simulink model "TST_InjCtl_qCo"  (R2016b)
settings: Solver=FixedStepDiscrete  StartTime=0.0  StopTime=simTime  FixedStep=sampleTime  RelTol=1e-3
values from neighbouring files (symbols this model uses):
  testCase = 1    [initTST_InjCtl_qCo_001.m]    (also in initTST_InjCtl_qCo_002.m = 2; initTST_InjCtl_qCo_003.m = 3; initTST_InjCtl_qCo_004.m = 4)
libraries: simulink x9, UnitTest_Lib x6
settings Model: Creator=zhengjinyan  LastModifiedBy=zhengjinyan
settings DebuggingCC: SignalRangeChecking=error

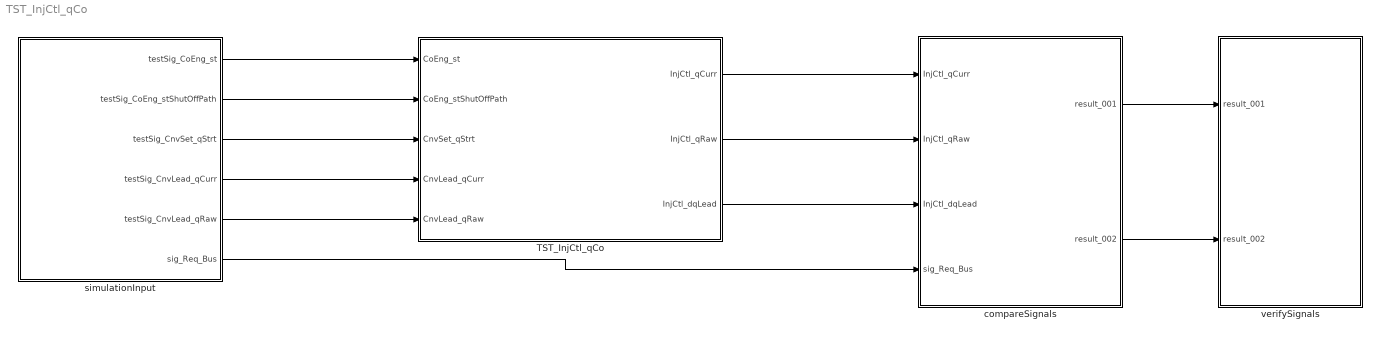
== system TST_InjCtl_qCo ==
  TST_InjCtl_qCo : Subsystem
  compareSignals : Subsystem
  simulationInput : Subsystem
  verifySignals : Subsystem
  wires:
  simulationInput/1(testSig_CoEng_st) -> TST_InjCtl_qCo/1(CoEng_st)
  simulationInput/2(testSig_CoEng_stShutOffPath) -> TST_InjCtl_qCo/2(CoEng_stShutOffPath)
  simulationInput/3(testSig_CnvSet_qStrt) -> TST_InjCtl_qCo/3(CnvSet_qStrt)
  simulationInput/4(testSig_CnvLead_qCurr) -> TST_InjCtl_qCo/4(CnvLead_qCurr)
  simulationInput/5(testSig_CnvLead_qRaw) -> TST_InjCtl_qCo/5(CnvLead_qRaw)
  TST_InjCtl_qCo/1(InjCtl_qCurr) -> compareSignals/1(InjCtl_qCurr)
  TST_InjCtl_qCo/2(InjCtl_qRaw) -> compareSignals/2(InjCtl_qRaw)
  TST_InjCtl_qCo/3(InjCtl_dqLead) -> compareSignals/3(InjCtl_dqLead)
  simulationInput/6(sig_Req_Bus) -> compareSignals/4(sig_Req_Bus)
  compareSignals/1(result_001) -> verifySignals/1(result_001)
  compareSignals/2(result_002) -> verifySignals/2(result_002)

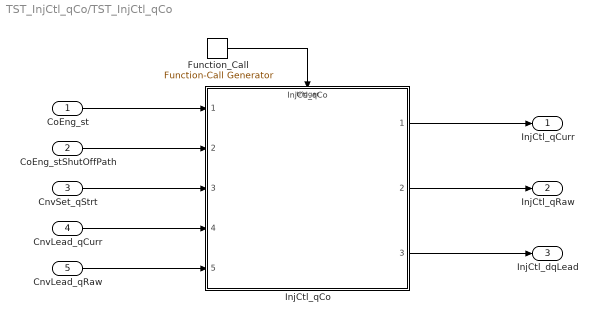
== system TST_InjCtl_qCo/TST_InjCtl_qCo ==
  CoEng_st : Inport
  CoEng_stShutOffPath : Inport  Port=2
  CnvSet_qStrt : Inport  Port=3
  CnvLead_qCurr : Inport  Port=4
  CnvLead_qRaw : Inport  Port=5
  Function_Call : simulink/Ports & Subsystems/Function-Call Generator  sample_time=sampleTime  numberOfIterations=1
  InjCtl_qCo : ModelReference  ModelNameDialog=InjCtl_qCo  SimulationMode=Normal  ModelReferenceVersion=1.10  TriggerPortName=function  TriggerPortTriggerType=function-call  TriggerPortStatesWhenEnabling=held
  InjCtl_qCurr : Outport
  InjCtl_qRaw : Outport  Port=2
  InjCtl_dqLead : Outport  Port=3
  wires:
  Function_Call/1 -> InjCtl_qCo/Trigger
  CoEng_st/1 -> InjCtl_qCo/1
  CoEng_stShutOffPath/1 -> InjCtl_qCo/2
  CnvSet_qStrt/1 -> InjCtl_qCo/3
  CnvLead_qCurr/1 -> InjCtl_qCo/4
  CnvLead_qRaw/1 -> InjCtl_qCo/5
  InjCtl_qCo/1 -> InjCtl_qCurr/1
  InjCtl_qCo/2 -> InjCtl_qRaw/1
  InjCtl_qCo/3 -> InjCtl_dqLead/1

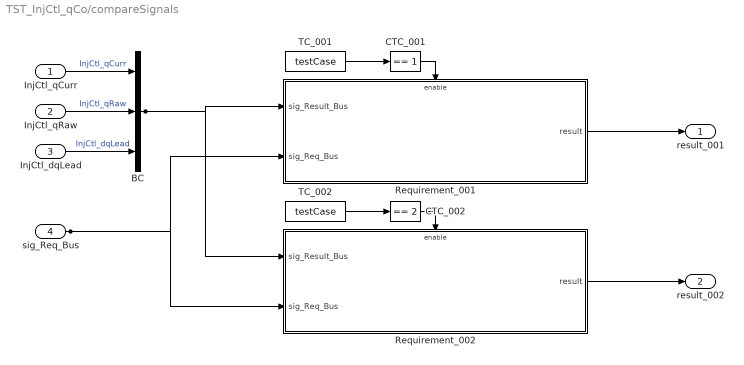
== system TST_InjCtl_qCo/compareSignals ==
  InjCtl_qCurr : Inport
  InjCtl_qRaw : Inport  Port=2
  InjCtl_dqLead : Inport  Port=3
  sig_Req_Bus : Inport  Port=4
  BC : BusCreator  Inputs=3
  CTC_001 : simulink/Logic and Bit Operations/Compare To Constant  relop===  const=1  OutDataTypeStr=boolean
  CTC_002 : simulink/Logic and Bit Operations/Compare To Constant  relop===  const=2  OutDataTypeStr=boolean
  Requirement_001 : Subsystem
  Requirement_002 : Subsystem
  TC_001 : Constant  Value=testCase
  TC_002 : Constant  Value=testCase
  result_001 : Outport
  result_002 : Outport  Port=2
  wires:
  InjCtl_qCurr/1 -> BC/1  "InjCtl_qCurr"
  InjCtl_qRaw/1 -> BC/2  "InjCtl_qRaw"
  InjCtl_dqLead/1 -> BC/3  "InjCtl_dqLead"
  TC_001/1 -> CTC_001/1
  CTC_001/1 -> Requirement_001/Enable
  sig_Req_Bus/1 -> Requirement_001/2(sig_Req_Bus), Requirement_002/2(sig_Req_Bus)
  BC/1 -> Requirement_001/1(sig_Result_Bus), Requirement_002/1(sig_Result_Bus)
  Requirement_001/1(result) -> result_001/1
  TC_002/1 -> CTC_002/1
  CTC_002/1 -> Requirement_002/Enable
  Requirement_002/1(result) -> result_002/1

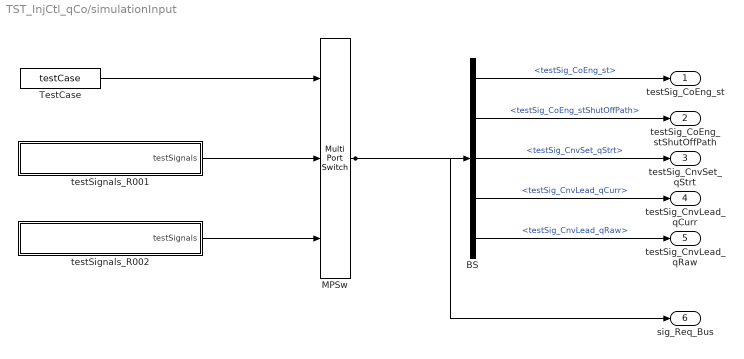
== system TST_InjCtl_qCo/simulationInput ==
  BS : BusSelector  OutputSignals=testSig_CoEng_st,testSig_CoEng_stShutOffPath,testSig_CnvSet_qStrt,testSig_CnvLead_qCurr,testSig_CnvLead_qRaw
  MPSw : MultiPortSwitch  Inputs=2  SaturateOnIntegerOverflow=on  InputSameDT=on
  TestCase : Constant  Value=testCase
  testSignals_R001 : Subsystem
  testSignals_R002 : Subsystem
  testSig_CoEng_st : Outport
  testSig_CoEng_stShutOffPath : Outport  Port=2
  testSig_CnvSet_qStrt : Outport  Port=3
  testSig_CnvLead_qCurr : Outport  Port=4
  testSig_CnvLead_qRaw : Outport  Port=5
  sig_Req_Bus : Outport  Port=6
  wires:
  BS/1 -> testSig_CoEng_st/1  "<testSig_CoEng_st>"
  BS/2 -> testSig_CoEng_stShutOffPath/1  "<testSig_CoEng_stShutOffPath>"
  BS/3 -> testSig_CnvSet_qStrt/1  "<testSig_CnvSet_qStrt>"
  BS/4 -> testSig_CnvLead_qCurr/1  "<testSig_CnvLead_qCurr>"
  BS/5 -> testSig_CnvLead_qRaw/1  "<testSig_CnvLead_qRaw>"
  MPSw/1 -> BS/1, sig_Req_Bus/1
  TestCase/1 -> MPSw/1
  testSignals_R001/1(testSignals) -> MPSw/2
  testSignals_R002/1(testSignals) -> MPSw/3

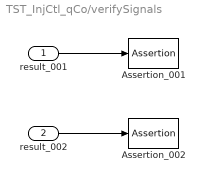
== system TST_InjCtl_qCo/verifySignals ==
  result_001 : Inport
  result_002 : Inport  Port=2
  Assertion_001 : Assertion  Enabled=off
  Assertion_002 : Assertion  Enabled=off
  wires:
  result_001/1 -> Assertion_001/1
  result_002/1 -> Assertion_002/1

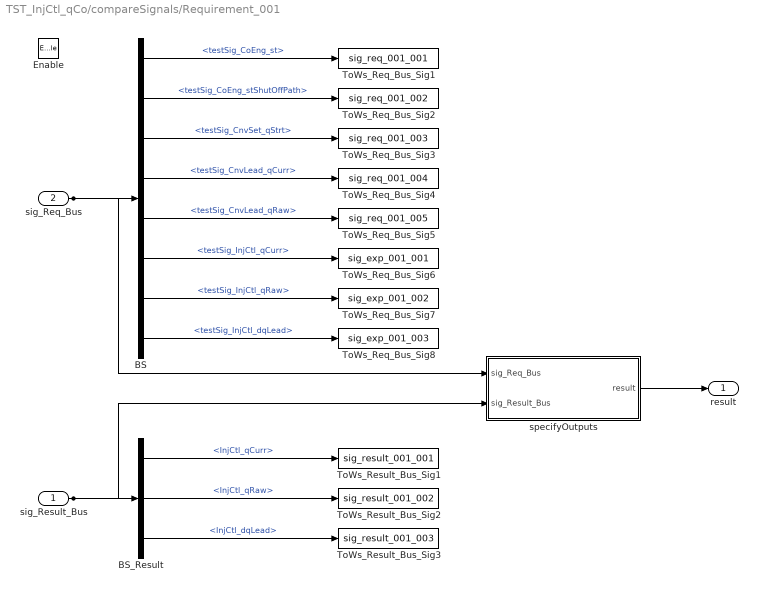
== system TST_InjCtl_qCo/compareSignals/Requirement_001 ==
  sig_Result_Bus : Inport
  sig_Req_Bus : Inport  Port=2
  Enable : EnablePort
  BS : BusSelector  OutputSignals=testSig_CoEng_st,testSig_CoEng_stShutOffPath,testSig_CnvSet_qStrt,testSig_CnvLead_qCurr,testSig_CnvLead_qRaw,testSig_InjCtl_qCurr,testSig_InjCtl_qRaw,testSig_InjCtl_dqLead
  BS_Result : BusSelector  OutputSignals=InjCtl_qCurr,InjCtl_qRaw,InjCtl_dqLead
  ToWs_Req_Bus_Sig1 : ToWorkspace  VariableName=sig_req_001_001  SaveFormat=Structure With Time
  ToWs_Req_Bus_Sig2 : ToWorkspace  VariableName=sig_req_001_002  SaveFormat=Structure With Time
  ToWs_Req_Bus_Sig3 : ToWorkspace  VariableName=sig_req_001_003  SaveFormat=Structure With Time
  ToWs_Req_Bus_Sig4 : ToWorkspace  VariableName=sig_req_001_004  SaveFormat=Structure With Time
  ToWs_Req_Bus_Sig5 : ToWorkspace  VariableName=sig_req_001_005  SaveFormat=Structure With Time
  ToWs_Req_Bus_Sig6 : ToWorkspace  VariableName=sig_exp_001_001  SaveFormat=Structure With Time
  ToWs_Req_Bus_Sig7 : ToWorkspace  VariableName=sig_exp_001_002  SaveFormat=Structure With Time
  ToWs_Req_Bus_Sig8 : ToWorkspace  VariableName=sig_exp_001_003  SaveFormat=Structure With Time
  ToWs_Result_Bus_Sig1 : ToWorkspace  VariableName=sig_result_001_001  SaveFormat=Structure With Time
  ToWs_Result_Bus_Sig2 : ToWorkspace  VariableName=sig_result_001_002  SaveFormat=Structure With Time
  ToWs_Result_Bus_Sig3 : ToWorkspace  VariableName=sig_result_001_003  SaveFormat=Structure With Time
  specifyOutputs : Subsystem
  result : Outport
  wires:
  sig_Req_Bus/1 -> BS/1, specifyOutputs/1(sig_Req_Bus)
  BS/1 -> ToWs_Req_Bus_Sig1/1  "<testSig_CoEng_st>"
  BS/2 -> ToWs_Req_Bus_Sig2/1  "<testSig_CoEng_stShutOffPath>"
  BS/3 -> ToWs_Req_Bus_Sig3/1  "<testSig_CnvSet_qStrt>"
  BS/4 -> ToWs_Req_Bus_Sig4/1  "<testSig_CnvLead_qCurr>"
  BS/5 -> ToWs_Req_Bus_Sig5/1  "<testSig_CnvLead_qRaw>"
  BS/6 -> ToWs_Req_Bus_Sig6/1  "<testSig_InjCtl_qCurr>"
  BS/7 -> ToWs_Req_Bus_Sig7/1  "<testSig_InjCtl_qRaw>"
  BS/8 -> ToWs_Req_Bus_Sig8/1  "<testSig_InjCtl_dqLead>"
  sig_Result_Bus/1 -> BS_Result/1, specifyOutputs/2(sig_Result_Bus)
  BS_Result/1 -> ToWs_Result_Bus_Sig1/1  "<InjCtl_qCurr>"
  BS_Result/2 -> ToWs_Result_Bus_Sig2/1  "<InjCtl_qRaw>"
  BS_Result/3 -> ToWs_Result_Bus_Sig3/1  "<InjCtl_dqLead>"
  specifyOutputs/1(result) -> result/1

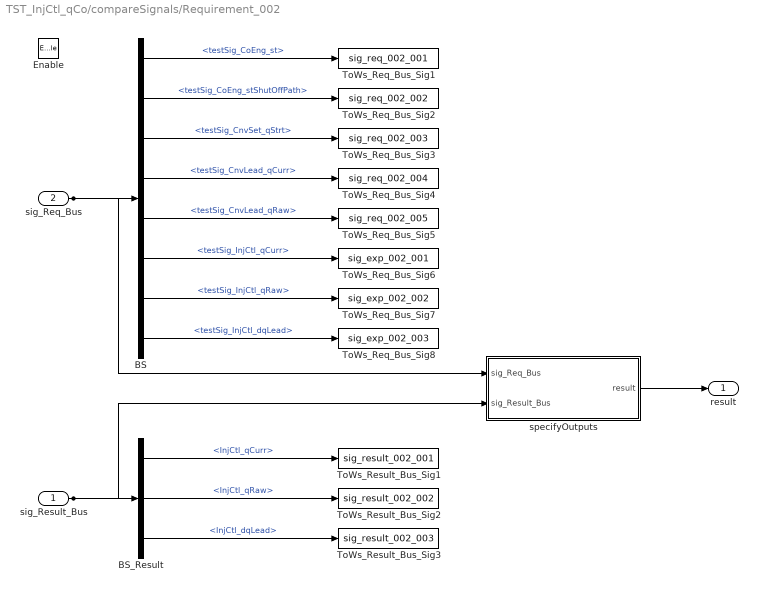
== system TST_InjCtl_qCo/compareSignals/Requirement_002 ==
  sig_Result_Bus : Inport
  sig_Req_Bus : Inport  Port=2
  Enable : EnablePort
  BS : BusSelector  OutputSignals=testSig_CoEng_st,testSig_CoEng_stShutOffPath,testSig_CnvSet_qStrt,testSig_CnvLead_qCurr,testSig_CnvLead_qRaw,testSig_InjCtl_qCurr,testSig_InjCtl_qRaw,testSig_InjCtl_dqLead
  BS_Result : BusSelector  OutputSignals=InjCtl_qCurr,InjCtl_qRaw,InjCtl_dqLead
  ToWs_Req_Bus_Sig1 : ToWorkspace  VariableName=sig_req_002_001  SaveFormat=Structure With Time
  ToWs_Req_Bus_Sig2 : ToWorkspace  VariableName=sig_req_002_002  SaveFormat=Structure With Time
  ToWs_Req_Bus_Sig3 : ToWorkspace  VariableName=sig_req_002_003  SaveFormat=Structure With Time
  ToWs_Req_Bus_Sig4 : ToWorkspace  VariableName=sig_req_002_004  SaveFormat=Structure With Time
  ToWs_Req_Bus_Sig5 : ToWorkspace  VariableName=sig_req_002_005  SaveFormat=Structure With Time
  ToWs_Req_Bus_Sig6 : ToWorkspace  VariableName=sig_exp_002_001  SaveFormat=Structure With Time
  ToWs_Req_Bus_Sig7 : ToWorkspace  VariableName=sig_exp_002_002  SaveFormat=Structure With Time
  ToWs_Req_Bus_Sig8 : ToWorkspace  VariableName=sig_exp_002_003  SaveFormat=Structure With Time
  ToWs_Result_Bus_Sig1 : ToWorkspace  VariableName=sig_result_002_001  SaveFormat=Structure With Time
  ToWs_Result_Bus_Sig2 : ToWorkspace  VariableName=sig_result_002_002  SaveFormat=Structure With Time
  ToWs_Result_Bus_Sig3 : ToWorkspace  VariableName=sig_result_002_003  SaveFormat=Structure With Time
  specifyOutputs : Subsystem
  result : Outport
  wires:
  sig_Req_Bus/1 -> BS/1, specifyOutputs/1(sig_Req_Bus)
  BS/1 -> ToWs_Req_Bus_Sig1/1  "<testSig_CoEng_st>"
  BS/2 -> ToWs_Req_Bus_Sig2/1  "<testSig_CoEng_stShutOffPath>"
  BS/3 -> ToWs_Req_Bus_Sig3/1  "<testSig_CnvSet_qStrt>"
  BS/4 -> ToWs_Req_Bus_Sig4/1  "<testSig_CnvLead_qCurr>"
  BS/5 -> ToWs_Req_Bus_Sig5/1  "<testSig_CnvLead_qRaw>"
  BS/6 -> ToWs_Req_Bus_Sig6/1  "<testSig_InjCtl_qCurr>"
  BS/7 -> ToWs_Req_Bus_Sig7/1  "<testSig_InjCtl_qRaw>"
  BS/8 -> ToWs_Req_Bus_Sig8/1  "<testSig_InjCtl_dqLead>"
  sig_Result_Bus/1 -> BS_Result/1, specifyOutputs/2(sig_Result_Bus)
  BS_Result/1 -> ToWs_Result_Bus_Sig1/1  "<InjCtl_qCurr>"
  BS_Result/2 -> ToWs_Result_Bus_Sig2/1  "<InjCtl_qRaw>"
  BS_Result/3 -> ToWs_Result_Bus_Sig3/1  "<InjCtl_dqLead>"
  specifyOutputs/1(result) -> result/1

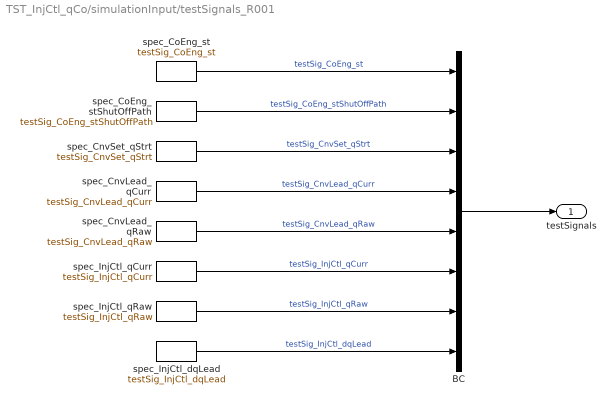
== system TST_InjCtl_qCo/simulationInput/testSignals_R001 ==
  BC : BusCreator  Inputs=8
  spec_CnvLead_qCurr : FromWorkspace  VariableName=testSig_CnvLead_qCurr  Interpolate=off  OutputAfterFinalValue=Holding final value
  spec_CnvLead_qRaw : FromWorkspace  VariableName=testSig_CnvLead_qRaw  Interpolate=off  OutputAfterFinalValue=Holding final value
  spec_CnvSet_qStrt : FromWorkspace  VariableName=testSig_CnvSet_qStrt  Interpolate=off  OutputAfterFinalValue=Holding final value
  spec_CoEng_st : FromWorkspace  VariableName=testSig_CoEng_st  Interpolate=off  OutputAfterFinalValue=Holding final value
  spec_CoEng_stShutOffPath : FromWorkspace  VariableName=testSig_CoEng_stShutOffPath  Interpolate=off  OutputAfterFinalValue=Holding final value
  spec_InjCtl_dqLead : FromWorkspace  VariableName=testSig_InjCtl_dqLead  Interpolate=off  OutputAfterFinalValue=Holding final value
  spec_InjCtl_qCurr : FromWorkspace  VariableName=testSig_InjCtl_qCurr  Interpolate=off  OutputAfterFinalValue=Holding final value
  spec_InjCtl_qRaw : FromWorkspace  VariableName=testSig_InjCtl_qRaw  Interpolate=off  OutputAfterFinalValue=Holding final value
  testSignals : Outport
  wires:
  BC/1 -> testSignals/1
  spec_CoEng_st/1 -> BC/1  "testSig_CoEng_st"
  spec_CoEng_stShutOffPath/1 -> BC/2  "testSig_CoEng_stShutOffPath"
  spec_CnvSet_qStrt/1 -> BC/3  "testSig_CnvSet_qStrt"
  spec_CnvLead_qCurr/1 -> BC/4  "testSig_CnvLead_qCurr"
  spec_CnvLead_qRaw/1 -> BC/5  "testSig_CnvLead_qRaw"
  spec_InjCtl_qCurr/1 -> BC/6  "testSig_InjCtl_qCurr"
  spec_InjCtl_qRaw/1 -> BC/7  "testSig_InjCtl_qRaw"
  spec_InjCtl_dqLead/1 -> BC/8  "testSig_InjCtl_dqLead"

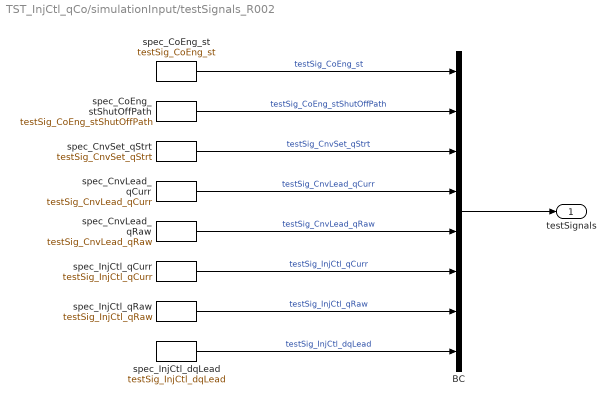
== system TST_InjCtl_qCo/simulationInput/testSignals_R002 ==
  BC : BusCreator  Inputs=8
  spec_CnvLead_qCurr : FromWorkspace  VariableName=testSig_CnvLead_qCurr  Interpolate=off  OutputAfterFinalValue=Holding final value
  spec_CnvLead_qRaw : FromWorkspace  VariableName=testSig_CnvLead_qRaw  Interpolate=off  OutputAfterFinalValue=Holding final value
  spec_CnvSet_qStrt : FromWorkspace  VariableName=testSig_CnvSet_qStrt  Interpolate=off  OutputAfterFinalValue=Holding final value
  spec_CoEng_st : FromWorkspace  VariableName=testSig_CoEng_st  Interpolate=off  OutputAfterFinalValue=Holding final value
  spec_CoEng_stShutOffPath : FromWorkspace  VariableName=testSig_CoEng_stShutOffPath  Interpolate=off  OutputAfterFinalValue=Holding final value
  spec_InjCtl_dqLead : FromWorkspace  VariableName=testSig_InjCtl_dqLead  Interpolate=off  OutputAfterFinalValue=Holding final value
  spec_InjCtl_qCurr : FromWorkspace  VariableName=testSig_InjCtl_qCurr  Interpolate=off  OutputAfterFinalValue=Holding final value
  spec_InjCtl_qRaw : FromWorkspace  VariableName=testSig_InjCtl_qRaw  Interpolate=off  OutputAfterFinalValue=Holding final value
  testSignals : Outport
  wires:
  BC/1 -> testSignals/1
  spec_CoEng_st/1 -> BC/1  "testSig_CoEng_st"
  spec_CoEng_stShutOffPath/1 -> BC/2  "testSig_CoEng_stShutOffPath"
  spec_CnvSet_qStrt/1 -> BC/3  "testSig_CnvSet_qStrt"
  spec_CnvLead_qCurr/1 -> BC/4  "testSig_CnvLead_qCurr"
  spec_CnvLead_qRaw/1 -> BC/5  "testSig_CnvLead_qRaw"
  spec_InjCtl_qCurr/1 -> BC/6  "testSig_InjCtl_qCurr"
  spec_InjCtl_qRaw/1 -> BC/7  "testSig_InjCtl_qRaw"
  spec_InjCtl_dqLead/1 -> BC/8  "testSig_InjCtl_dqLead"

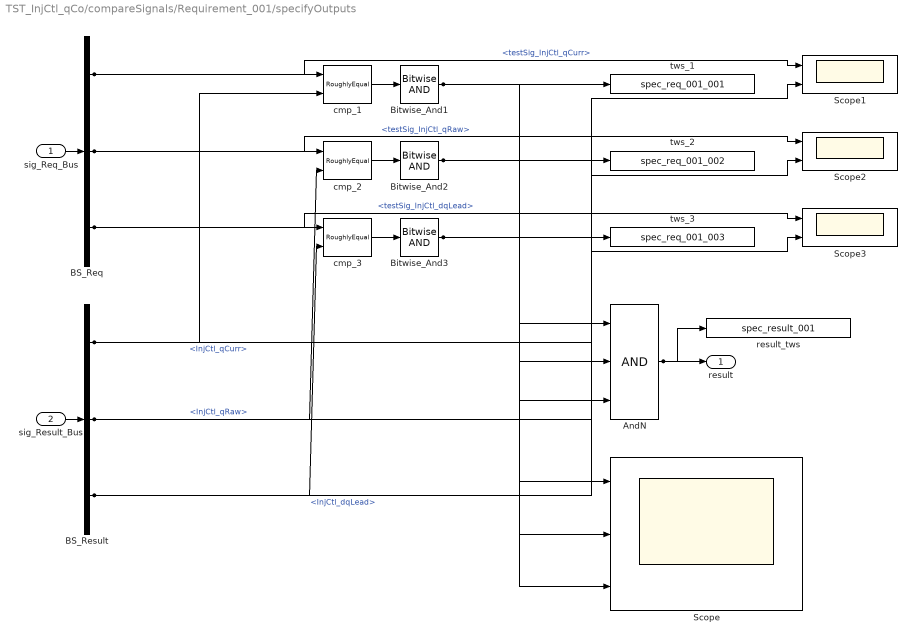
== system TST_InjCtl_qCo/compareSignals/Requirement_001/specifyOutputs ==
  sig_Req_Bus : Inport
  sig_Result_Bus : Inport  Port=2
  AndN : Logic  Inputs=3
  BS_Req : BusSelector  OutputSignals=testSig_InjCtl_qCurr,testSig_InjCtl_qRaw,testSig_InjCtl_dqLead
  BS_Result : BusSelector  OutputSignals=InjCtl_qCurr,InjCtl_qRaw,InjCtl_dqLead
  Bitwise_And1 : simulink/Logic and Bit Operations/Bitwise Operator  logicop=AND  UseBitMask=off  BitMask=bin2dec('11011001')  BitMaskRealWorld=Stored Integer
  Bitwise_And2 : simulink/Logic and Bit Operations/Bitwise Operator  logicop=AND  UseBitMask=off  BitMask=bin2dec('11011001')  BitMaskRealWorld=Stored Integer
  Bitwise_And3 : simulink/Logic and Bit Operations/Bitwise Operator  logicop=AND  UseBitMask=off  BitMask=bin2dec('11011001')  BitMaskRealWorld=Stored Integer
  Scope : Scope  NumInputPorts=3
  Scope1 : Scope  NumInputPorts=2
  Scope2 : Scope  NumInputPorts=2
  Scope3 : Scope  NumInputPorts=2
  cmp_1 : UnitTest_Lib/RoughlyEqual  slope=0.1
  cmp_2 : UnitTest_Lib/RoughlyEqual  slope=0.1
  cmp_3 : UnitTest_Lib/RoughlyEqual  slope=0.1
  result_tws : ToWorkspace  VariableName=spec_result_001
  tws_1 : ToWorkspace  VariableName=spec_req_001_001
  tws_2 : ToWorkspace  VariableName=spec_req_001_002
  tws_3 : ToWorkspace  VariableName=spec_req_001_003
  result : Outport
  wires:
  sig_Req_Bus/1 -> BS_Req/1
  sig_Result_Bus/1 -> BS_Result/1
  AndN/1 -> result/1, result_tws/1
  BS_Req/1 -> cmp_1/1, Scope1/1  "<testSig_InjCtl_qCurr>"
  BS_Result/1 -> cmp_1/2, Scope1/2  "<InjCtl_qCurr>"
  cmp_1/1 -> Bitwise_And1/1
  Bitwise_And1/1 -> tws_1/1, AndN/1, Scope/1
  BS_Req/2 -> cmp_2/1, Scope2/1  "<testSig_InjCtl_qRaw>"
  BS_Result/2 -> cmp_2/2, Scope2/2  "<InjCtl_qRaw>"
  cmp_2/1 -> Bitwise_And2/1
  Bitwise_And2/1 -> tws_2/1, AndN/2, Scope/2
  BS_Req/3 -> cmp_3/1, Scope3/1  "<testSig_InjCtl_dqLead>"
  BS_Result/3 -> cmp_3/2, Scope3/2  "<InjCtl_dqLead>"
  cmp_3/1 -> Bitwise_And3/1
  Bitwise_And3/1 -> tws_3/1, AndN/3, Scope/3

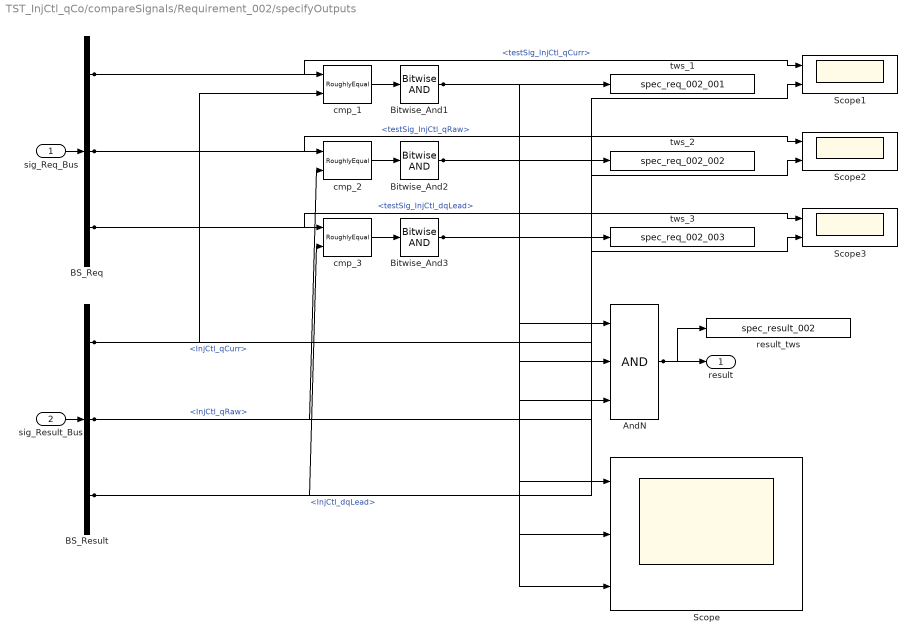
== system TST_InjCtl_qCo/compareSignals/Requirement_002/specifyOutputs ==
  sig_Req_Bus : Inport
  sig_Result_Bus : Inport  Port=2
  AndN : Logic  Inputs=3
  BS_Req : BusSelector  OutputSignals=testSig_InjCtl_qCurr,testSig_InjCtl_qRaw,testSig_InjCtl_dqLead
  BS_Result : BusSelector  OutputSignals=InjCtl_qCurr,InjCtl_qRaw,InjCtl_dqLead
  Bitwise_And1 : simulink/Logic and Bit Operations/Bitwise Operator  logicop=AND  UseBitMask=off  BitMask=bin2dec('11011001')  BitMaskRealWorld=Stored Integer
  Bitwise_And2 : simulink/Logic and Bit Operations/Bitwise Operator  logicop=AND  UseBitMask=off  BitMask=bin2dec('11011001')  BitMaskRealWorld=Stored Integer
  Bitwise_And3 : simulink/Logic and Bit Operations/Bitwise Operator  logicop=AND  UseBitMask=off  BitMask=bin2dec('11011001')  BitMaskRealWorld=Stored Integer
  Scope : Scope  NumInputPorts=3
  Scope1 : Scope  NumInputPorts=2
  Scope2 : Scope  NumInputPorts=2
  Scope3 : Scope  NumInputPorts=2
  cmp_1 : UnitTest_Lib/RoughlyEqual  slope=0.1
  cmp_2 : UnitTest_Lib/RoughlyEqual  slope=0.1
  cmp_3 : UnitTest_Lib/RoughlyEqual  slope=0.1
  result_tws : ToWorkspace  VariableName=spec_result_002
  tws_1 : ToWorkspace  VariableName=spec_req_002_001
  tws_2 : ToWorkspace  VariableName=spec_req_002_002
  tws_3 : ToWorkspace  VariableName=spec_req_002_003
  result : Outport
  wires:
  sig_Req_Bus/1 -> BS_Req/1
  sig_Result_Bus/1 -> BS_Result/1
  AndN/1 -> result/1, result_tws/1
  BS_Req/1 -> cmp_1/1, Scope1/1  "<testSig_InjCtl_qCurr>"
  BS_Result/1 -> cmp_1/2, Scope1/2  "<InjCtl_qCurr>"
  cmp_1/1 -> Bitwise_And1/1
  Bitwise_And1/1 -> tws_1/1, AndN/1, Scope/1
  BS_Req/2 -> cmp_2/1, Scope2/1  "<testSig_InjCtl_qRaw>"
  BS_Result/2 -> cmp_2/2, Scope2/2  "<InjCtl_qRaw>"
  cmp_2/1 -> Bitwise_And2/1
  Bitwise_And2/1 -> tws_2/1, AndN/2, Scope/2
  BS_Req/3 -> cmp_3/1, Scope3/1  "<testSig_InjCtl_dqLead>"
  BS_Result/3 -> cmp_3/2, Scope3/2  "<InjCtl_dqLead>"
  cmp_3/1 -> Bitwise_And3/1
  Bitwise_And3/1 -> tws_3/1, AndN/3, Scope/3
